simulink model "SST_v2_21b"  (R2021b)
settings: Solver=ode1be  StartTime=0.0  StopTime=1  FixedStep=Ts  RelTol=1e-3
values from neighbouring files (symbols this model uses):
  Kiv = 1/Tpv    (= 22527.3933103)    [DC_Grid_Light.m]
  Kpv = Tzv/Tpv    (= 0.187728277586)    [DC_Grid_Light.m]
undefined symbols (not defined in the file or in its folder): Cout, Imax, Kii, Kpi, Lfilter, Lgrid, Rfilter, Rgrid, RLoad, Ts, VAC_pk
libraries: simulink x62, spsVoltageMeasurementLib x21, spsParallelRLCBranchLib x15, spsFullBridgeConverterLib x15, spsACVoltageSourceLib x3, spsCurrentMeasurementLib x3, spsGroundLib x3, slpidlib x3, spsSeriesRLCBranchLib x3, spspowerguiLib x1
(part 2 of 2)

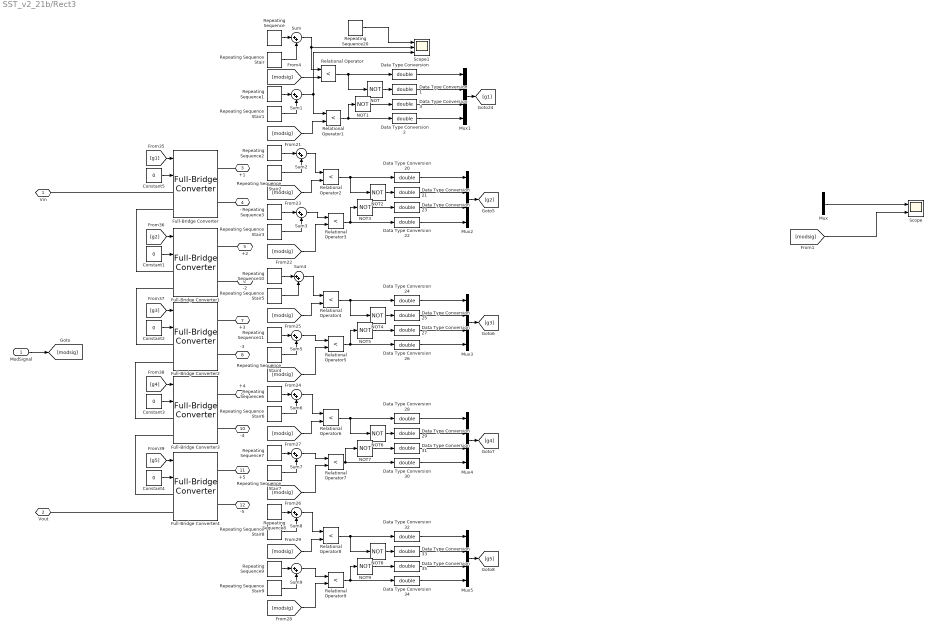
== system SST_v2_21b/Rect3 ==
  ModSignal : Inport
  Constant{1..5} (5 alike) : Constant  Value=0
  Data Type Conversion{,1..3,20..35} (20 alike) : DataTypeConversion  OutMin=[0]  OutMax=[1]  OutDataTypeStr=double
  Full-Bridge Converter{,1..4} (5 alike) : spsFullBridgeConverterLib/Full-Bridge Converter  ModelType=Switching devices  Ron=Rdson  Rs=Rsnubber  Cs=Csnubber  Vforward=[0,0]  Ron_Diode=1e-3  Rs_Diode=1e6  Cs_Diode=inf  Vf_Diode=1e-3  Rs_CurrentSource=inf
      settings: SourceProductBaseCode=PS
  Mux : Mux  Inputs=10
  Mux{1..5} (5 alike) : Mux
  NOT{,1..9} (10 alike) : Logic  Operator=NOT  IconShape=distinctive  AllPortsSameDT=off  OutDataTypeStr=boolean
  Relational Operator{,1..9} (10 alike) : RelationalOperator  Operator=<  OutDataTypeStr=boolean  RndMeth=Simplest
  Repeating Sequence : simulink/Sources/Repeating Sequence  rep_seq_t=Tcarriers  rep_seq_y=Ac11
  Repeating Sequence Stair : simulink/Sources/Repeating Sequence Stair  OutValues=Sc11  tsamp=TswS  OutMin=[]  OutMax=[]  OutDataTypeStr=double  OutputDataTypeScalingMode=double  OutDataType=fixdt(0,8)  ConRadixGroup=Best Precision: Vector-wise  OutScaling=2^-12
  Repeating Sequence Stair1 : simulink/Sources/Repeating Sequence Stair  OutValues=Sc12  tsamp=TswS  OutMin=[]  OutMax=[]  OutDataTypeStr=double  OutputDataTypeScalingMode=double  OutDataType=fixdt(0,8)  ConRadixGroup=Best Precision: Vector-wise  OutScaling=2^-12
  Repeating Sequence Stair2 : simulink/Sources/Repeating Sequence Stair  OutValues=Sc21  tsamp=TswS  OutMin=[]  OutMax=[]  OutDataTypeStr=double  OutputDataTypeScalingMode=double  OutDataType=fixdt(0,8)  ConRadixGroup=Best Precision: Vector-wise  OutScaling=2^-12
  Repeating Sequence Stair3 : simulink/Sources/Repeating Sequence Stair  OutValues=Sc22  tsamp=TswS  OutMin=[]  OutMax=[]  OutDataTypeStr=double  OutputDataTypeScalingMode=double  OutDataType=fixdt(0,8)  ConRadixGroup=Best Precision: Vector-wise  OutScaling=2^-12
  Repeating Sequence Stair4 : simulink/Sources/Repeating Sequence Stair  OutValues=Sc32  tsamp=TswS  OutMin=[]  OutMax=[]  OutDataTypeStr=double  OutputDataTypeScalingMode=double  OutDataType=fixdt(0,8)  ConRadixGroup=Best Precision: Vector-wise  OutScaling=2^-12
  Repeating Sequence Stair5 : simulink/Sources/Repeating Sequence Stair  OutValues=Sc31  tsamp=TswS  OutMin=[]  OutMax=[]  OutDataTypeStr=double  OutputDataTypeScalingMode=double  OutDataType=fixdt(0,8)  ConRadixGroup=Best Precision: Vector-wise  OutScaling=2^-12
  Repeating Sequence Stair6 : simulink/Sources/Repeating Sequence Stair  OutValues=Sc41  tsamp=TswS  OutMin=[]  OutMax=[]  OutDataTypeStr=double  OutputDataTypeScalingMode=double  OutDataType=fixdt(0,8)  ConRadixGroup=Best Precision: Vector-wise  OutScaling=2^-12
  Repeating Sequence Stair7 : simulink/Sources/Repeating Sequence Stair  OutValues=Sc42  tsamp=TswS  OutMin=[]  OutMax=[]  OutDataTypeStr=double  OutputDataTypeScalingMode=double  OutDataType=fixdt(0,8)  ConRadixGroup=Best Precision: Vector-wise  OutScaling=2^-12
  Repeating Sequence Stair8 : simulink/Sources/Repeating Sequence Stair  OutValues=Sc51  tsamp=TswS  OutMin=[]  OutMax=[]  OutDataTypeStr=double  OutputDataTypeScalingMode=double  OutDataType=fixdt(0,8)  ConRadixGroup=Best Precision: Vector-wise  OutScaling=2^-12
  Repeating Sequence Stair9 : simulink/Sources/Repeating Sequence Stair  OutValues=Sc52  tsamp=TswS  OutMin=[]  OutMax=[]  OutDataTypeStr=double  OutputDataTypeScalingMode=double  OutDataType=fixdt(0,8)  ConRadixGroup=Best Precision: Vector-wise  OutScaling=2^-12
  Repeating Sequence1 : simulink/Sources/Repeating Sequence  rep_seq_t=Tcarriers  rep_seq_y=AC12
  Repeating Sequence10 : simulink/Sources/Repeating Sequence  rep_seq_t=Tcarriers  rep_seq_y=Ac31
  Repeating Sequence11 : simulink/Sources/Repeating Sequence  rep_seq_t=Tcarriers  rep_seq_y=AC32
  Repeating Sequence2 : simulink/Sources/Repeating Sequence  rep_seq_t=Tcarriers  rep_seq_y=Ac21
  Repeating Sequence20 : simulink/Sources/Repeating Sequence  rep_seq_t=Tcarriers  rep_seq_y=Ac11
  Repeating Sequence3 : simulink/Sources/Repeating Sequence  rep_seq_t=Tcarriers  rep_seq_y=Ac22
  Repeating Sequence6 : simulink/Sources/Repeating Sequence  rep_seq_t=Tcarriers  rep_seq_y=Ac41
  Repeating Sequence7 : simulink/Sources/Repeating Sequence  rep_seq_t=Tcarriers  rep_seq_y=Ac42
  Repeating Sequence8 : simulink/Sources/Repeating Sequence  rep_seq_t=Tcarriers  rep_seq_y=Ac51
  Repeating Sequence9 : simulink/Sources/Repeating Sequence  rep_seq_t=Tcarriers  rep_seq_y=Ac52
  Scope : Scope  NumInputPorts=2
  Scope1 : Scope  NumInputPorts=3
  Sum{,1..9} (10 alike) : Sum  Inputs=|++
  Vin : PMIOPort  Side=Left
  Vout : PMIOPort  Port=2  Side=Left
  +1 : PMIOPort  Port=3  Side=Right
  -1 : PMIOPort  Port=4  Side=Right
  +2 : PMIOPort  Port=5  Side=Right
  -2 : PMIOPort  Port=6  Side=Right
  +3 : PMIOPort  Port=7  Side=Right
  -3 : PMIOPort  Port=8  Side=Right
  +4 : PMIOPort  Port=9  Side=Right
  -4 : PMIOPort  Port=10  Side=Right
  +5 : PMIOPort  Port=11  Side=Right
  -5 : PMIOPort  Port=12  Side=Right
  wires:
  Data Type Conversion/1 -> Mux1/1
  [modsig] -> Relational Operator7/2
  Data Type Conversion33/1 -> Mux5/2
  NOT2/1 -> Data Type Conversion21/1
  Data Type Conversion30/1 -> Mux4/4
  Constant5/1 -> Full-Bridge Converter/2
  Data Type Conversion31/1 -> Mux4/3
  Data Type Conversion23/1 -> Mux2/3
  [g4] -> Full-Bridge Converter3/1
  NOT8/1 -> Data Type Conversion33/1
  Constant4/1 -> Full-Bridge Converter4/2
  Data Type Conversion29/1 -> Mux4/2
  Data Type Conversion24/1 -> Mux3/1
  Data Type Conversion25/1 -> Mux3/2
  NOT7/1 -> Data Type Conversion31/1
  Mux5/1 -> [g5]
  [g1] -> Full-Bridge Converter/1
  NOT5/1 -> Data Type Conversion27/1
  NOT3/1 -> Data Type Conversion23/1
  Relational Operator8/1 -> Data Type Conversion32/1, NOT8/1
  Data Type Conversion26/1 -> Mux3/4
  [modsig] -> Relational Operator6/2
  Relational Operator3/1 -> Data Type Conversion22/1, NOT3/1
  Mux1/1 -> [g1]
  Constant2/1 -> Full-Bridge Converter2/2
  Data Type Conversion3/1 -> Mux1/3
  Mux4/1 -> [g4]
  Relational Operator5/1 -> Data Type Conversion26/1, NOT5/1
  Relational Operator1/1 -> Data Type Conversion2/1, NOT1/1
  Constant1/1 -> Full-Bridge Converter1/2
  [modsig] -> Relational Operator3/2
  Relational Operator/1 -> Data Type Conversion/1, NOT/1
  [g2] -> Full-Bridge Converter1/1
  Mux2/1 -> [g2]
  Relational Operator4/1 -> Data Type Conversion24/1, NOT4/1
  [modsig] -> Relational Operator/2
  [modsig] -> Relational Operator9/2
  Data Type Conversion32/1 -> Mux5/1
  NOT/1 -> Data Type Conversion1/1
  Data Type Conversion35/1 -> Mux5/3
  Relational Operator6/1 -> Data Type Conversion28/1, NOT6/1
  [modsig] -> Relational Operator1/2
  NOT6/1 -> Data Type Conversion29/1
  NOT1/1 -> Data Type Conversion3/1
  [modsig] -> Relational Operator5/2
  Data Type Conversion21/1 -> Mux2/2
  Data Type Conversion27/1 -> Mux3/3
  Relational Operator2/1 -> Data Type Conversion20/1, NOT2/1
  Mux3/1 -> [g3]
  Relational Operator7/1 -> Data Type Conversion30/1, NOT7/1
  Data Type Conversion34/1 -> Mux5/4
  [modsig] -> Relational Operator4/2
  NOT9/1 -> Data Type Conversion35/1
  [g3] -> Full-Bridge Converter2/1
  Data Type Conversion28/1 -> Mux4/1
  Data Type Conversion20/1 -> Mux2/1
  Repeating Sequence3/1 -> Sum3/1
  [modsig] -> Relational Operator2/2
  Relational Operator9/1 -> Data Type Conversion34/1, NOT9/1
  [modsig] -> Relational Operator8/2
  Constant3/1 -> Full-Bridge Converter3/2
  Data Type Conversion1/1 -> Mux1/2
  NOT4/1 -> Data Type Conversion25/1
  Data Type Conversion2/1 -> Mux1/4
  Data Type Conversion22/1 -> Mux2/4
  [g5] -> Full-Bridge Converter4/1
  ModSignal/1 -> [modsig]
  Mux/1 -> Scope/1
  [modsig] -> Scope/2
  Repeating Sequence/1 -> Sum/1
  Sum/1 -> Scope1/2, Relational Operator/1
  Repeating Sequence1/1 -> Sum1/1
  Repeating Sequence Stair1/1 -> Sum1/2
  Sum1/1 -> Scope1/3, Relational Operator1/1
  Repeating Sequence2/1 -> Sum2/1
  Repeating Sequence Stair2/1 -> Sum2/2
  Sum2/1 -> Relational Operator2/1
  Sum3/1 -> Relational Operator3/1
  Repeating Sequence Stair3/1 -> Sum3/2
  Repeating Sequence10/1 -> Sum4/1
  Repeating Sequence Stair5/1 -> Sum4/2
  Sum4/1 -> Relational Operator4/1
  Repeating Sequence11/1 -> Sum5/1
  Sum5/1 -> Relational Operator5/1
  Repeating Sequence Stair4/1 -> Sum5/2
  Repeating Sequence6/1 -> Sum6/1
  Repeating Sequence Stair6/1 -> Sum6/2
  Sum6/1 -> Relational Operator6/1
  Repeating Sequence7/1 -> Sum7/1
  Repeating Sequence Stair7/1 -> Sum7/2
  Sum7/1 -> Relational Operator7/1
  Repeating Sequence8/1 -> Sum8/1
  Sum8/1 -> Relational Operator8/1
  Repeating Sequence Stair8/1 -> Sum8/2
  Repeating Sequence9/1 -> Sum9/1
  Repeating Sequence Stair9/1 -> Sum9/2
  Sum9/1 -> Relational Operator9/1
  Repeating Sequence20/1 -> Scope1/1
  Repeating Sequence Stair/1 -> Sum/2
  connections:
  Full-Bridge Converter2/LConn2 -- Full-Bridge Converter3/LConn1
  +3/RConn1 -- Full-Bridge Converter2/RConn1
  -2/RConn1 -- Full-Bridge Converter1/RConn2
  Full-Bridge Converter1/LConn2 -- Full-Bridge Converter2/LConn1
  Full-Bridge Converter4/LConn2 -- Vout/RConn1
  +1/RConn1 -- Full-Bridge Converter/RConn1
  Full-Bridge Converter/LConn1 -- Vin/RConn1
  -4/RConn1 -- Full-Bridge Converter3/RConn2
  -1/RConn1 -- Full-Bridge Converter/RConn2
  +4/RConn1 -- Full-Bridge Converter3/RConn1
  -3/RConn1 -- Full-Bridge Converter2/RConn2
  Full-Bridge Converter4/LConn1 -- Full-Bridge Converter3/LConn2
  +5/RConn1 -- Full-Bridge Converter4/RConn1
  +2/RConn1 -- Full-Bridge Converter1/RConn1
  -5/RConn1 -- Full-Bridge Converter4/RConn2
  Full-Bridge Converter/LConn2 -- Full-Bridge Converter1/LConn1

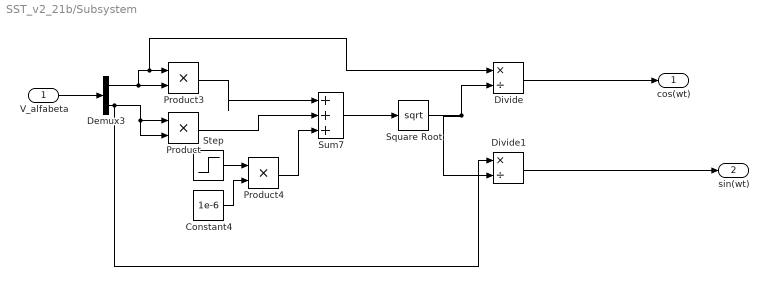
== system SST_v2_21b/Subsystem ==
  V_alfabeta : Inport
  Constant4 : Constant  Value=1e-6
  Demux3 : Demux  Outputs=2
  Divide : Product  Inputs=*/
  Divide1 : Product  Inputs=*/
  Product : Product
  Product3 : Product
  Product4 : Product
  Square Root : Sqrt  SaturateOnIntegerOverflow=on
  Step : Step  Time=Ts  Before=1  After=0  SampleTime=0
  Sum7 : Sum  Inputs=|+++
  cos(wt) : Outport
  sin(wt) : Outport  Port=2
  wires:
  Divide1/1 -> sin(wt)/1
  Demux3/2 -> Product/2, Product/1, Divide1/1
  Product3/1 -> Sum7/1
  Product/1 -> Sum7/2
  Constant4/1 -> Product4/2
  Square Root/1 -> Divide1/2, Divide/2
  V_alfabeta/1 -> Demux3/1
  Product4/1 -> Sum7/3
  Demux3/1 -> Product3/2, Divide/1, Product3/1
  Divide/1 -> cos(wt)/1
  Sum7/1 -> Square Root/1
  Step/1 -> Product4/1

== matlab function SST_v2_21b/MATLAB Function ==
  data: abc3 input; alfabeta2 output
function alfabeta2  = fcn( abc3)
alfabeta2 = [0.8164965809277259 -0.4082482904638631 -0.4082482904638631;0 0.7071067811865475 -0.7071067811865475]*abc3;
end

== matlab function SST_v2_21b/MATLAB Function2 ==
  data: abc3 input; alfabeta2 output
function alfabeta2  = fcn( abc3)
alfabeta2 = [0.8164965809277259 -0.4082482904638631 -0.4082482904638631;0 0.7071067811865475 -0.7071067811865475]*abc3;
end

== matlab function SST_v2_21b/MATLAB Function3 ==
  data: alfabeta input; dq2 output; cossinwt input
function dq2  = fcn( alfabeta,cossinwt)
dq2 = [cossinwt(1) cossinwt(2);-cossinwt(2) cossinwt(1)]*alfabeta;
end

== matlab function SST_v2_21b/MATLAB Function4 ==
  data: dq input; alfabeta output; cossinwt input
function alfabeta  = fcn(dq,cossinwt)
alfabeta = [cossinwt(1) -cossinwt(2);cossinwt(2) cossinwt(1)]*dq;
end

== matlab function SST_v2_21b/MATLAB Function5 ==
  data: alfabeta2 input; abc3 output
function abc3  = fcn(alfabeta2)
abc3 = [0.8164965809277259 0; -0.4082482904638631 0.7071067811865476; -0.4082482904638631 -0.7071067811865475]*alfabeta2;
end

== matlab function SST_v2_21b/MATLAB Function1 ==
  data: alfabeta input; dq2 output; cossinwt input
function dq2  = fcn( alfabeta,cossinwt)
dq2 = [cossinwt(1) cossinwt(2);-cossinwt(2) cossinwt(1)]*alfabeta;
end
